simulink model "task1_2"  (R2022b)
settings: Solver=VariableStepAuto  StartTime=0.0  StopTime=10  RelTol=1e-3
values from neighbouring files (symbols this model uses):
  C = 1e-06    [task1_2m.mat]    (also in task1_3m.mat)
  R = 1000000    [task1_2m.mat]    (also in task1_3m.mat)
settings Model: Creator=faraz  LastModifiedBy=faraz

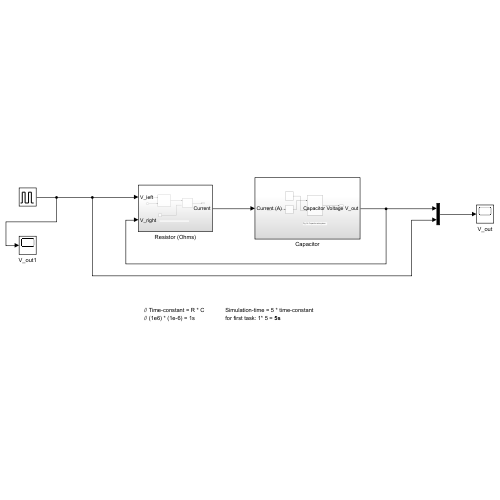
[thumbnail: Simulink's stored preview of the top-level diagram]
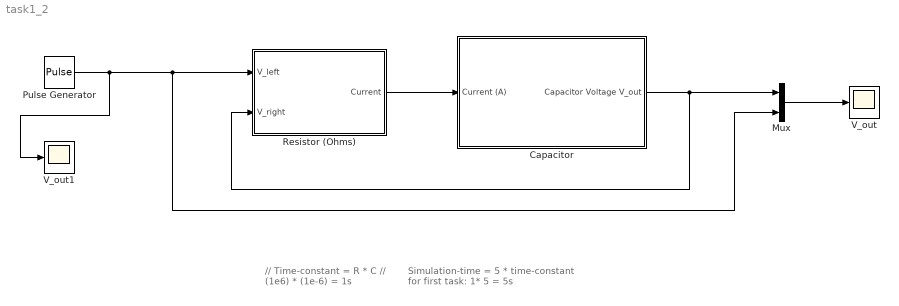
== system task1_2 ==
  note: Simulation-time = 5 * time-constant
      | for first task: 1* 5 = 5s
  note: // Time-constant = R * C
      | // (1e6) * (1e-6) = 1s
  Capacitor : Subsystem
  Mux : Mux  Inputs=2
  Pulse Generator : DiscretePulseGenerator  PulseType=Time based  Period=10  PulseWidth=50
  Resistor (Ohms) : Subsystem
  V_out : Scope
  V_out1 : Scope
  wires:
  Resistor (Ohms)/1(Current) -> Capacitor/1(Current (A))
  Mux/1 -> V_out/1
  Capacitor/1(Capacitor Voltage V_out) -> Mux/1, Resistor (Ohms)/2(V_right)
  Pulse Generator/1 -> V_out1/1, Mux/2, Resistor (Ohms)/1(V_left)

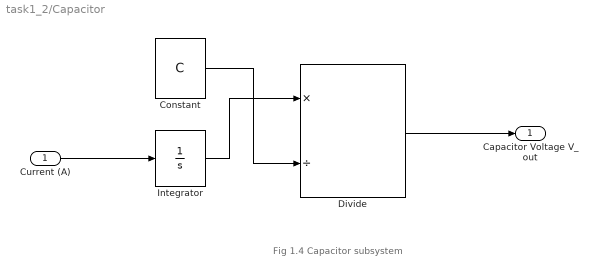
== system task1_2/Capacitor ==
  note: Fig 1.4 Capacitor subsystem
  Current (A) : Inport
  Constant : Constant  Value=C
  Divide : Product  Inputs=*/
  Integrator : Integrator  InitialCondition=1
  Capacitor Voltage V_out : Outport
  wires:
  Divide/1 -> Capacitor Voltage V_out/1
  Integrator/1 -> Divide/1
  Constant/1 -> Divide/2
  Current (A)/1 -> Integrator/1

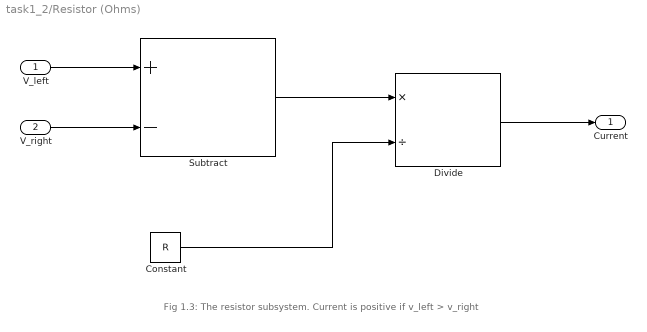
== system task1_2/Resistor (Ohms) ==
  note: Fig 1.3: The resistor subsystem. Current is positive if v_left > v_right
  V_left : Inport
  V_right : Inport  Port=2
  Constant : Constant  Value=R
  Divide : Product  Inputs=*/
  Subtract : Sum  Inputs=+-
  Current : Outport
  wires:
  Constant/1 -> Divide/2
  Subtract/1 -> Divide/1
  Divide/1 -> Current/1
  V_left/1 -> Subtract/1
  V_right/1 -> Subtract/2
